simulink model "Questao_3"  (R2023b)
settings: Solver=VariableStepAuto  StartTime=0.0  StopTime=20  RelTol=1e-3
settings Model: Creator=pedro  LastModifiedBy=pedro

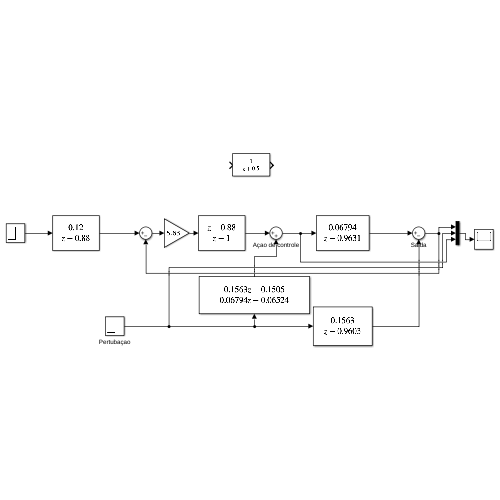
[thumbnail: Simulink's stored preview of the top-level diagram]
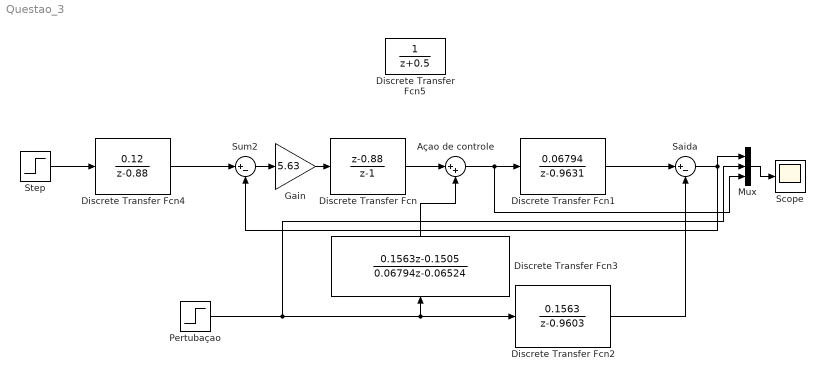
== system Questao_3 ==
  Açao de controle : Sum  Inputs=|++
  Discrete Transfer Fcn : DiscreteTransferFcn  Numerator=[1 -0.88]  Denominator=[1 -1]
  Discrete Transfer Fcn1 : DiscreteTransferFcn  Numerator=[0.06794]  Denominator=[1 -0.9631]
  Discrete Transfer Fcn2 : DiscreteTransferFcn  Numerator=[0.1563]  Denominator=[1 -0.9603]
  Discrete Transfer Fcn3 : DiscreteTransferFcn  Numerator=[0.1563 -0.1505]  Denominator=[0.06794 -0.06524]
  Discrete Transfer Fcn4 : DiscreteTransferFcn  Numerator=[0.12]  Denominator=[1 -0.88]
  Discrete Transfer Fcn5 : DiscreteTransferFcn
  Gain : Gain  Gain=5.63
  Mux : Mux  Inputs=3
  Pertubaçao : Step  Time=10  SampleTime=0.162
  Saida : Sum  Inputs=|+-
  Scope : Scope
  Step : Step  SampleTime=0.162
  Sum2 : Sum  Inputs=|+-
  wires:
  Discrete Transfer Fcn/1 -> Açao de controle/1
  Açao de controle/1 -> Mux/3, Discrete Transfer Fcn1/1
  Discrete Transfer Fcn1/1 -> Saida/1
  Discrete Transfer Fcn2/1 -> Saida/2
  Pertubaçao/1 -> Mux/2, Discrete Transfer Fcn2/1, Discrete Transfer Fcn3/1
  Saida/1 -> Sum2/2, Mux/1
  Mux/1 -> Scope/1
  Gain/1 -> Discrete Transfer Fcn/1
  Sum2/1 -> Gain/1
  Step/1 -> Discrete Transfer Fcn4/1
  Discrete Transfer Fcn4/1 -> Sum2/1
  Discrete Transfer Fcn3/1 -> Açao de controle/2
